simulink model "ModelloTeam1"  (R2022b)
settings: Solver=VariableStepAuto  StartTime=0.0  StopTime=120  RelTol=1e-3
settings Model: Creator=giova  LastModifiedBy=giova

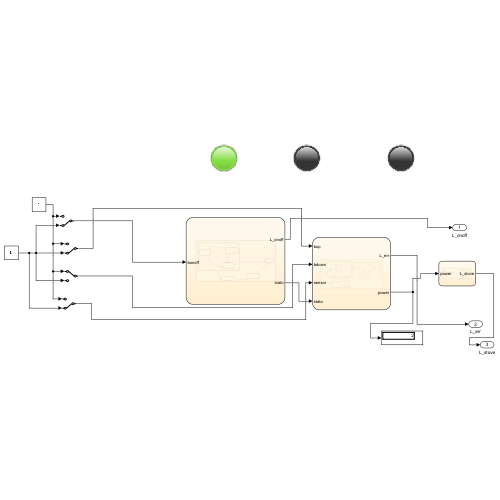
[thumbnail: Simulink's stored preview of the top-level diagram]
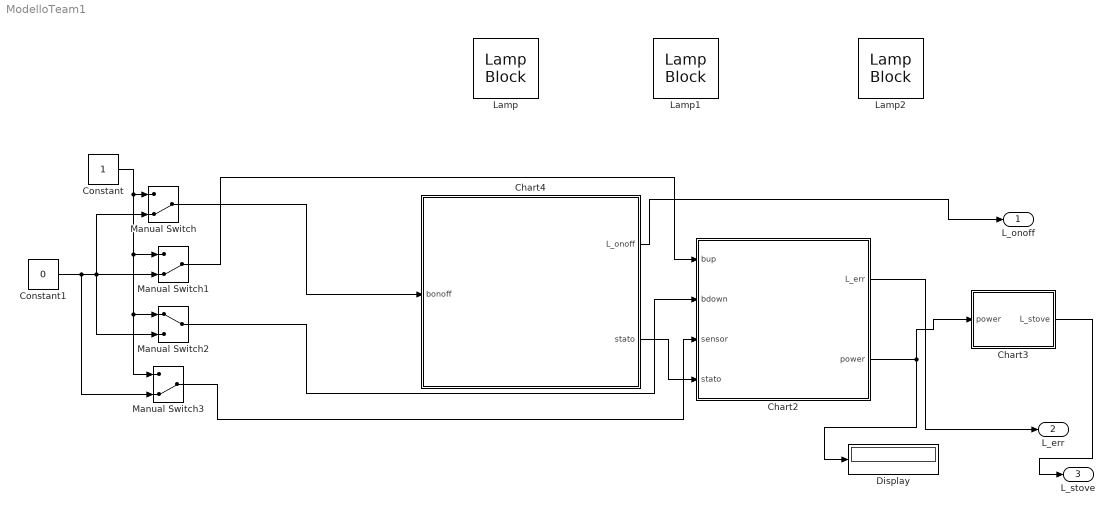
== system ModelloTeam1 ==
  Chart2 : Stateflow chart  TreatAsAtomicUnit=on
  Chart3 : Stateflow chart  TreatAsAtomicUnit=on
  Chart4 : Stateflow chart  TreatAsAtomicUnit=on
  Constant : Constant
  Constant1 : Constant  Value=0
  Display : Display
  Lamp : LampBlock  LabelPosition=Hide
  Lamp1 : LampBlock  LabelPosition=Hide
  Lamp2 : LampBlock  LabelPosition=Hide
  Manual Switch : ManualSwitch  CurrentSetting=0
  Manual Switch1 : ManualSwitch  CurrentSetting=0
  Manual Switch2 : ManualSwitch
  Manual Switch3 : ManualSwitch  CurrentSetting=0
  L_onoff : Outport
  L_err : Outport  Port=2
  L_stove : Outport  Port=3
  wires:
  Chart4/2(stato) -> Chart2/4(stato)
  Chart2/2(power) -> Chart3/1(power), Display/1
  Constant/1 -> Manual Switch3/1, Manual Switch2/1, Manual Switch1/1, Manual Switch/1
  Constant1/1 -> Manual Switch3/2, Manual Switch2/2, Manual Switch1/2, Manual Switch/2
  Manual Switch/1 -> Chart4/1(bonoff)
  Manual Switch1/1 -> Chart2/1(bup)
  Manual Switch2/1 -> Chart2/2(bdown)
  Manual Switch3/1 -> Chart2/3(sensor)
  Chart4/1(L_onoff) -> L_onoff/1
  Chart2/1(L_err) -> L_err/1
  Chart3/1(L_stove) -> L_stove/1

== stateflow chart ModelloTeam1/Chart2 ==
  settings: updateMethod=DISCRETE  sampleTime=0.25
  state Power_and_error_management
    state Power_management [parallel]
      settings: executionOrder=1
      state PowerUD_manager_on
        state PowerUp
          en: temp_power=temp_power/2
        state Check_buttons
          en: power=temp_power;
        state PowerDown
          en: temp_power=temp_power*2
        PowerUp -> Check_buttons [order 4] : [power==MAX_TIMING & sensor~=ACTIVE]{temp_power=MAX_TIMING}
        PowerUp -> Check_buttons [order 2] : after(TIMER,sec)
        Check_buttons -> PowerUp [order 1] : [power~=MIN_TIMING  & bup_second==PRESSED]
        PowerUp -> PowerUp [order 3] : [temp_power~=MIN_TIMING  & bup_second==PRESSED]
        PowerUp -> PowerDown [order 1] : [bdown_second==PRESSED]
        PowerDown -> PowerUp [order 1] : [ bup_second==PRESSED]
        (default) -> Check_buttons
        Check_buttons -> PowerDown [order 2] : [power~=MAX_TIMING & bdown_second==PRESSED]
        PowerDown -> Check_buttons [order 4] : [power==MAX_TIMING & sensor~=ACTIVE]{temp_power=MAX_TIMING}
        PowerDown -> Check_buttons [order 2] : after(TIMER,sec)
        PowerDown -> PowerDown [order 3] : [temp_power~=MAX_TIMING & bdown_second==PRESSED]
      state PowerUD_manager_off
        en: temp_power=MAX_TIMING
        power=MAX_TIMING;
      (default) -> PowerUD_manager_off
      PowerUD_manager_off -> PowerUD_manager_on : [stato==ON]
      PowerUD_manager_on -> PowerUD_manager_off : [stato==OFF]
    state Button_up_down_management [parallel]
      settings: executionOrder=2
      state Button_up_down_manager_on
        state Longpressed_DOWN_button
          en: bdown_second = RELEASED;
        state Longpressed_UP_botton
          en: bup_second = RELEASED;
        state Pressed_DOWN_button
          en: bdown_second = RELEASED;
          on after(BUTTONDURATION,sec):
          bdown_second=PRESSED;
        state Pressed_UP_botton
          en: bup_second = RELEASED;
          on after(BUTTONDURATION,sec):
          bup_second=PRESSED;
        state Wait_Up_Down_button
          en: bup_second=RELEASED;
          bdown_second=RELEASED;
        Longpressed_UP_botton -> Wait_Up_Down_button : [bup==RELEASED]
        Pressed_UP_botton -> Longpressed_UP_botton [order 2] : [bup_second==PRESSED & bup == PRESSED]
        Pressed_DOWN_button -> Longpressed_DOWN_button [order 1] : [bdown_second==PRESSED & bdown == PRESSED]
        Longpressed_DOWN_button -> Wait_Up_Down_button : [bdown==RELEASED]
        Pressed_UP_botton -> Wait_Up_Down_button [order 1] : [bup==RELEASED | sensor ~=ACTIVE]
        Pressed_DOWN_button -> Wait_Up_Down_button [order 2] : [bdown==RELEASED | sensor~=ACTIVE]
        Wait_Up_Down_button -> Pressed_UP_botton [order 2] : [bup==PRESSED & sensor==ACTIVE]
        (default) -> Wait_Up_Down_button
        Wait_Up_Down_button -> Pressed_DOWN_button [order 1] : [bdown==PRESSED & sensor==ACTIVE]
      state Button_up_down_manager_off
      Button_up_down_manager_off -> Button_up_down_manager_on : [stato==ON]
      Button_up_down_manager_on -> Button_up_down_manager_off : [stato==OFF]
      (default) -> Button_up_down_manager_off
    state Error_management [parallel]
      settings: executionOrder=3
      state Error_manager_on
        state Wait_blinking
          en: power=MAX_TIMING;
          temp_power=MAX_TIMING;
        state Check_error
        state Start_error
          en: L_err=ON;
          ex: L_err =OFF;
        (default) -> Wait_blinking
        Check_error -> Wait_blinking [order 2] : [power==MAX_TIMING]
        Wait_blinking -> Check_error : [power<MAX_TIMING]
        Start_error -> Check_error [order 1] : [sensor==ACTIVE]
        Check_error -> Start_error [order 1] : [sensor~=ACTIVE]
        Start_error -> Wait_blinking [order 2] : after(ERR_TIMER,sec)
      state Error_manager_off
        en: L_err=OFF;
      Error_manager_off -> Error_manager_on : [stato==ON]
      (default) -> Error_manager_off
      Error_manager_on -> Error_manager_off : [stato==OFF]
  (default) -> Power_and_error_management
  data: bup input; bdown input; sensor input; L_err output; RELEASED local =true; PRESSED local =false; BUTTONDURATION local =1; bup_second local; bdown_second local; ACTIVE local =0; ERR_TIMER local =10; ON local =true; OFF local =false; TIMER local =5; temp_power local; power output; stato input boolean; MAX_TIMING local =4; MIN_TIMING local =0.25

== stateflow chart ModelloTeam1/Chart3 ==
  settings: updateMethod=DISCRETE  sampleTime=0.25
  state Stove_management
    state Blinking_stove
      state Led_on
        en: L_stove=ON;
      state Led_off
        en: L_stove = OFF;
      (default) -> Led_on
      Led_off -> Led_on : after(power,sec)
      Led_on -> Led_off : after(power,sec)
    state Starting_power
      en: L_stove=OFF;
    (default) -> Starting_power
    Blinking_stove -> Starting_power : [power==MAX_TIMING]
    Starting_power -> Blinking_stove : [power<MAX_TIMING]
  data: ON local =true; OFF local =false; L_stove output; power input; MAX_TIMING local =4

== stateflow chart ModelloTeam1/Chart4 ==
  settings: updateMethod=DISCRETE  sampleTime=0.25
  state PowerOFF_management
    state PowerOFF_manager_on
      state Pressed_OFF_button
        en: bonoff_second = RELEASED;
        on after(BUTTONDURATION,sec):
        bonoff_second=PRESSED;
      state Longpressed_OFF_button
        en: bonoff_second = RELEASED
      state Wait_OFF_button
        en: bonoff_second=RELEASED;
      Pressed_OFF_button -> Longpressed_OFF_button [order 1] : [bonoff_second==PRESSED & bonoff == PRESSED]
      Wait_OFF_button -> Pressed_OFF_button : [bonoff == PRESSED]
      Pressed_OFF_button -> Wait_OFF_button [order 2] : [bonoff==RELEASED]
      Longpressed_OFF_button -> Wait_OFF_button : [bonoff == RELEASED]
      (default) -> Wait_OFF_button
    state W_post_power_off
      en: L_onoff=OFF;
      stato=OFF;
    state PowerOFF_manager_off
      en: stato=OFF;
      L_onoff=OFF;
    state W_post_power_on
      en: stato=ON;
      L_onoff=ON;
    PowerOFF_manager_on -> W_post_power_off : [bonoff_second==PRESSED]
    W_post_power_off -> PowerOFF_manager_off : [bonoff==RELEASED]
    W_post_power_on -> PowerOFF_manager_on : [bonoff==RELEASED]
    (default) -> PowerOFF_manager_off
    PowerOFF_manager_off -> W_post_power_on : [bonoff==PRESSED]
  data: L_onoff output; bonoff input; RELEASED local =true; PRESSED local =false; bonoff_second local; ON local =true; OFF local =false; BUTTONDURATION local =1; stato output
